simulink model "guitar2"  (Simulink 8.0)
settings: Solver=ode5  StartTime=0.0  StopTime=inf  FixedStep=0.001  RelTol=1e-3
libraries: simulink x4, xpclib x4, xpcnilib x4
settings Model: Creator=research account  LastModifiedBy=Admin  SimulationMode=external  BufferReuse=off
settings DataIOCC: SignalLoggingSaveFormat=ModelDataLogs
settings OptimizationCC: BlockReduction=off  OptimizeBlockIOStorage=off  BufferReuse=off  ExpressionFolding=off  LocalBlockOutputs=off
settings DebuggingCC: SingleTaskRateTransMsg=warning  FcnCallInpInsideContextMsg=UseLocalSettings  StrictBusMsg=Warning
settings HardwareCC: ProdIntDivRoundTo=Zero  ProdEndianess=LittleEndian  ProdHWDeviceType=Generic->32-bit x86 compatible
settings SFSimCC: SimParseCustomCode=off
settings RTWCC: SystemTargetFile=xpctarget.tlc  TemplateMakefile=xpc_default_tmf  Description=xPC Target  ProcessScript=xpctarget_make_rtw_hook  RTWCompilerOptimization=On
settings xpcTargetCC: TargetFcnLib=ansi_tfl_table_tmw.mat  CodeReplacementLibrary=XPC_BLAS  ParMdlRefBuildCompliant=on  ConcurrentExecutionCompliant=on  CombineSignalStateStructs=off  GRTInterface=on  xPCTaskExecutionProfile=off  xPCRL32EventNumber=5000  xpcObjCom=on  xPCLoadParamSetFile=off  xPCConcurrentTasks=off  xPCEnableSFAnimation=off

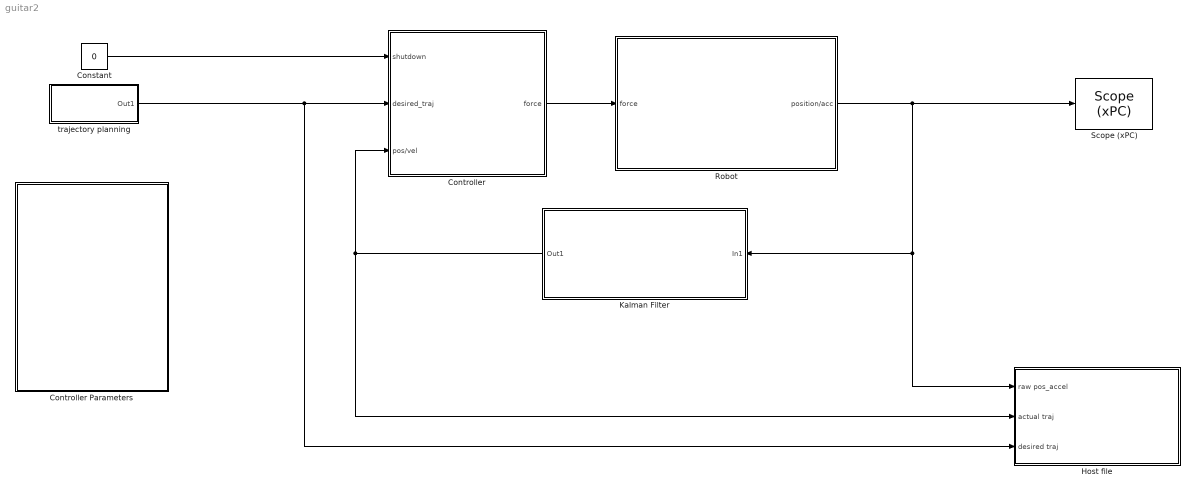
== system guitar2 ==
  Constant : Constant  Description=xPCTag(1) = onSwitch;  Value=0
  Controller : Subsystem
  Controller Parameters : Subsystem
      mask Display: disp('Controller Parameters')
  Host file : Subsystem
  Kalman Filter : Subsystem
  Robot : Subsystem
  "Scope (xPC) " : xpclib/Misc./Scope (xPC)   scopeno=1  scopetype=Target  autostart=on  viewmode=Graphical redraw  formatstr='%15.6f'  grid=on  ylimits=[0,0]  nosamples=500  noprepostsamples=0  interleave=1  triggermode=FreeRun  triggersignal=1  triggerlevel=0.0  triggerslope=Either  triggerscope=1  triggersample=0  filename=data.dat  mode=Lazy  writesize=512  autorestart=off  dynamicfilemode=off  maxwritefilesize=512*1024^2
  trajectory planning : Subsystem
  wires:
  Robot/1(position/acc) -> "Scope (xPC) "/1, Host file/1(raw pos_accel), Kalman Filter/1(In1)
  Constant/1 -> Controller/1(shutdown)
  Controller/1(force) -> Robot/1(force)
  trajectory planning/1(Out1) -> Controller/2(desired_traj), Host file/3(desired traj)
  Kalman Filter/1(Out1) -> Host file/2(actual traj), Controller/3(pos/vel)

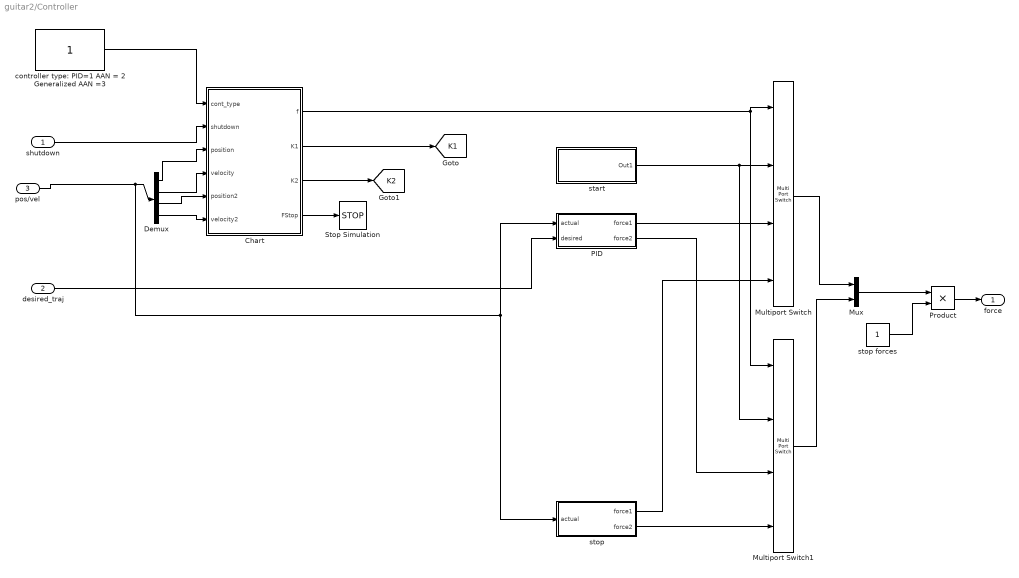
== system guitar2/Controller ==
  shutdown : Inport
  desired_traj : Inport  Port=2
  pos/vel : Inport  Port=3
  Chart : Stateflow chart  TreatAsAtomicUnit=on
  Demux : Demux
  Multiport Switch : MultiPortSwitch
  Multiport Switch1 : MultiPortSwitch
  Mux : Mux  Inputs=2
  PID : Subsystem
  Product : Product  RndMeth=Zero
  Stop Simulation : Stop
  controller type: PID=1 AAN = 2 Generalized AAN =3 : Constant
  start : Subsystem
  stop : Subsystem
  stop forces : Constant  Description=xPCTag(1) = stopForces;
  force : Outport
  tag scope: K1=global, K2=global
  wires:
  shutdown/1 -> Chart/2(shutdown)
  pos/vel/1 -> Demux/1, PID/1(actual), stop/1(actual)
  Demux/1 -> Chart/3(position)
  Demux/2 -> Chart/4(velocity)
  Chart/4(FStop) -> Stop Simulation/1
  controller type: PID=1 AAN = 2 Generalized AAN =3/1 -> Chart/1(cont_type)
  desired_traj/1 -> PID/2(desired)
  Chart/2(K1) -> [K1]
  Chart/3(K2) -> [K2]
  Demux/3 -> Chart/5(position2)
  Demux/4 -> Chart/6(velocity2)
  Mux/1 -> Product/1
  Product/1 -> force/1
  stop forces/1 -> Product/2
  Chart/1(f) -> Multiport Switch/1, Multiport Switch1/1
  start/1(Out1) -> Multiport Switch/2, Multiport Switch1/2
  PID/1(force1) -> Multiport Switch/3
  Multiport Switch/1 -> Mux/1
  PID/2(force2) -> Multiport Switch1/3
  stop/1(force1) -> Multiport Switch/4
  Multiport Switch1/1 -> Mux/2
  stop/2(force2) -> Multiport Switch1/4

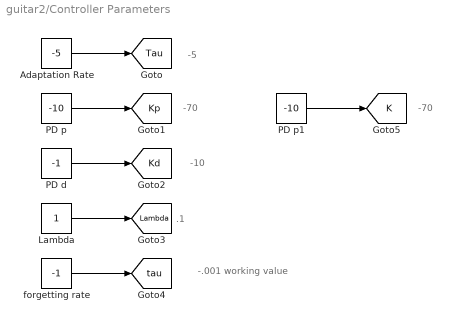
== system guitar2/Controller Parameters ==
  note: -.001 working value
  note: .1
  note: -10
  note: -70
  note: -5
  note: -70
  Adaptation Rate : Constant  Description=xPCTag(1)=learning_rate;  Value=-5
  Lambda : Constant
  PD d : Constant  Value=-1
  PD p : Constant  Value=-10
  PD p1 : Constant  Value=-10
  forgetting rate : Constant  Description=xPCTag(1)=forgetting_rate;  Value=-1
  tag scope: K=global, Kd=global, Kp=global, Lambda=global, Tau=global, tau=global
  wires:
  Adaptation Rate/1 -> [Tau]
  PD p/1 -> [Kp]
  PD d/1 -> [Kd]
  Lambda/1 -> [Lambda]
  forgetting rate/1 -> [tau]
  PD p1/1 -> [K]

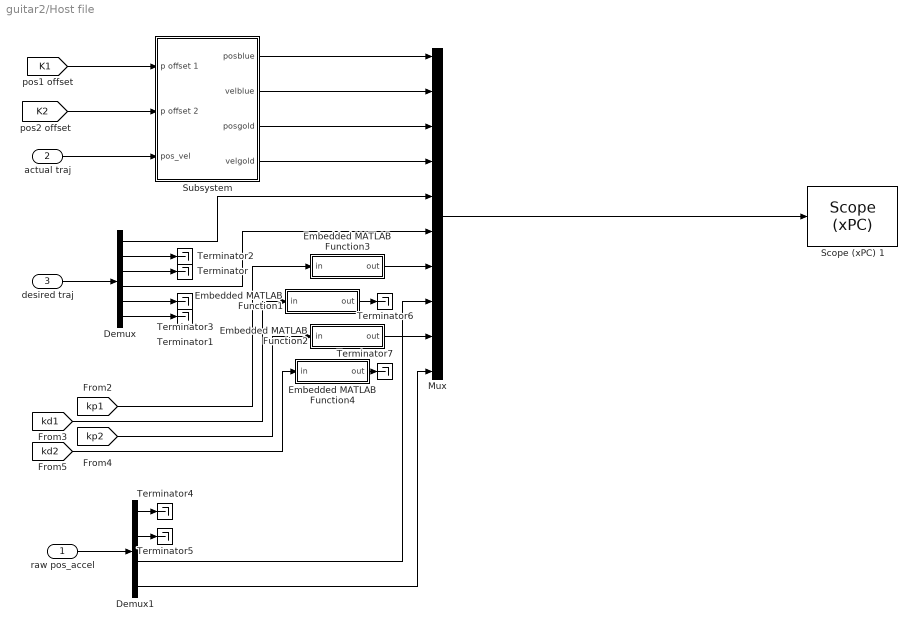
== system guitar2/Host file ==
  raw pos_accel : Inport
  actual traj : Inport  Port=2
  desired traj : Inport  Port=3
  Demux : Demux  Outputs=6
  Demux1 : Demux
  Embedded MATLAB Function1 : MATLAB Function  TreatAsAtomicUnit=on
  Embedded MATLAB Function2 : MATLAB Function  TreatAsAtomicUnit=on
  Embedded MATLAB Function3 : MATLAB Function  TreatAsAtomicUnit=on
  Embedded MATLAB Function4 : MATLAB Function  TreatAsAtomicUnit=on
  Mux : Mux  Inputs=10
  Scope (xPC) 1 : xpclib/Misc./Scope (xPC)   scopeno=3  scopetype=Host  autostart=on  viewmode=Graphical redraw  formatstr='%15.6f'  grid=on  ylimits=[0,0]  nosamples=500  noprepostsamples=0  interleave=1  triggermode=FreeRun  triggersignal=1  triggerlevel=0.0  triggerslope=Either  triggerscope=1  triggersample=0  filename=data.dat  mode=Lazy  writesize=512  autorestart=off  dynamicfilemode=off  maxwritefilesize=512*1024^2
  Subsystem : Subsystem
  Terminator{,1..7} (8 alike) : Terminator
  wires:
  desired traj/1 -> Demux/1
  Demux/3 -> Terminator/1
  Demux/6 -> Terminator1/1
  Demux/2 -> Terminator2/1
  Demux/5 -> Terminator3/1
  actual traj/1 -> Subsystem/3(pos_vel)
  [K1] -> Subsystem/1(p offset 1)
  [K2] -> Subsystem/2(p offset 2)
  Subsystem/1(posblue) -> Mux/1
  Subsystem/2(velblue) -> Mux/2
  Subsystem/3(posgold) -> Mux/3
  Subsystem/4(velgold) -> Mux/4
  Demux/1 -> Mux/5
  Demux/4 -> Mux/6
  [kp1] -> Embedded MATLAB Function3/1(in)
  [kd1] -> Embedded MATLAB Function1/1(in)
  [kp2] -> Embedded MATLAB Function2/1(in)
  [kd2] -> Embedded MATLAB Function4/1(in)
  Mux/1 -> Scope (xPC) 1/1
  Embedded MATLAB Function3/1(out) -> Mux/7
  Embedded MATLAB Function2/1(out) -> Mux/9
  raw pos_accel/1 -> Demux1/1
  Demux1/4 -> Mux/10
  Demux1/1 -> Terminator4/1
  Embedded MATLAB Function1/1(out) -> Terminator6/1
  Embedded MATLAB Function4/1(out) -> Terminator7/1
  Demux1/2 -> Terminator5/1
  Demux1/3 -> Mux/8

== system guitar2/Kalman Filter ==
  note: positions and velocities tagged here!
  In1 : Inport
  Demux : Demux
  Gain : Gain
  Mux : Mux  Inputs=2
  kalman1 : Subsystem
  kalman2 : Subsystem
  kalman3 : Subsystem
  kalman4 : Subsystem
  Out1 : Outport
  wires:
  Demux/1 -> kalman3/1(position)
  Demux/2 -> kalman4/1(position)
  Demux/3 -> kalman3/2(acc)
  Demux/4 -> kalman4/2(acc)
  In1/1 -> Demux/1
  kalman3/1(position/est_vel) -> Mux/1
  kalman4/1(position/est_vel) -> Mux/2
  Mux/1 -> Gain/1
  Gain/1 -> Out1/1

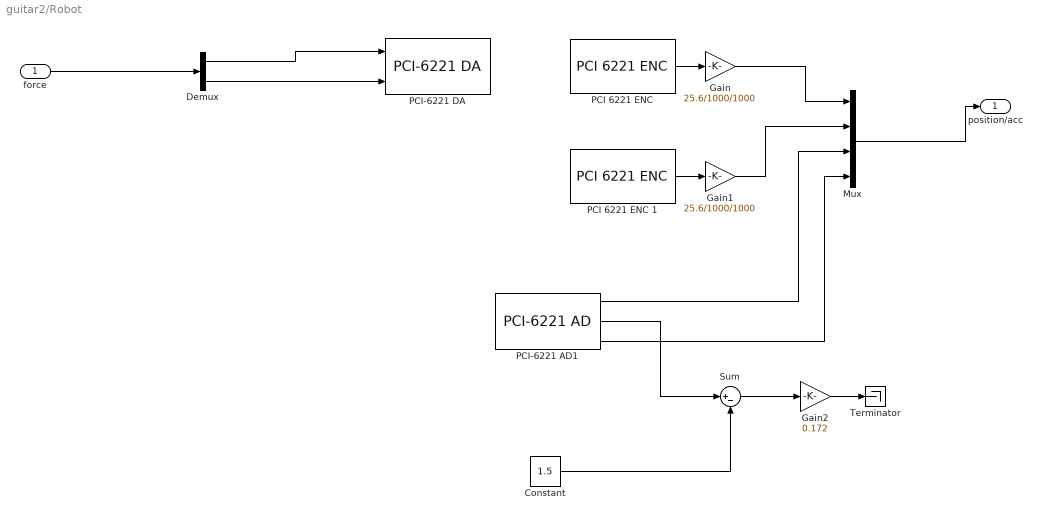
== system guitar2/Robot ==
  force : Inport
  Constant : Constant  Value=1.5
  Demux : Demux  Outputs=2
  Gain : Gain  Gain=25.6/1000/1000
  Gain1 : Gain  Gain=25.6/1000/1000
  Gain2 : Gain  Gain=0.172
  Mux : Mux
  "PCI 6221 ENC " : xpcnilib/Incremental Encoder/PCI 6221 ENC   channel=0  countMode=Quadrature Mode x4  initCount=0  reload=off  indexPhase=A low B low  filter=Minimum pulse width 125 nanoseconds  sampleTime=0.001  slot=-1
  PCI 6221 ENC 1 : xpcnilib/Incremental Encoder/PCI 6221 ENC   channel=1  countMode=Quadrature Mode x4  initCount=0  reload=off  indexPhase=A low B low  filter=Minimum pulse width 125 nanoseconds  sampleTime=0.001  slot=-1
  PCI-6221 AD1 : xpcnilib/A//D/M Series/PCI-6221 AD  channel=[1 2 3]  range=[10]  coupling=[0]  scantime=5e-6  sampletime=0.001  slot=-1
  PCI-6221 DA : xpcnilib/D//A/M Series/PCI-6221 DA  channel=[1 2]  reset=[1]  initValue=[0]  sampletime=0.001  slot=-1
  Sum : Sum  Inputs=|+-
  Terminator : Terminator
  position/acc : Outport
  wires:
  "PCI 6221 ENC "/1 -> Gain/1
  Gain/1 -> Mux/1
  Mux/1 -> position/acc/1
  Demux/1 -> PCI-6221 DA/1
  Demux/2 -> PCI-6221 DA/2
  force/1 -> Demux/1
  PCI 6221 ENC 1/1 -> Gain1/1
  Gain1/1 -> Mux/2
  PCI-6221 AD1/1 -> Mux/3
  PCI-6221 AD1/3 -> Mux/4
  PCI-6221 AD1/2 -> Sum/1
  Constant/1 -> Sum/2
  Sum/1 -> Gain2/1
  Gain2/1 -> Terminator/1

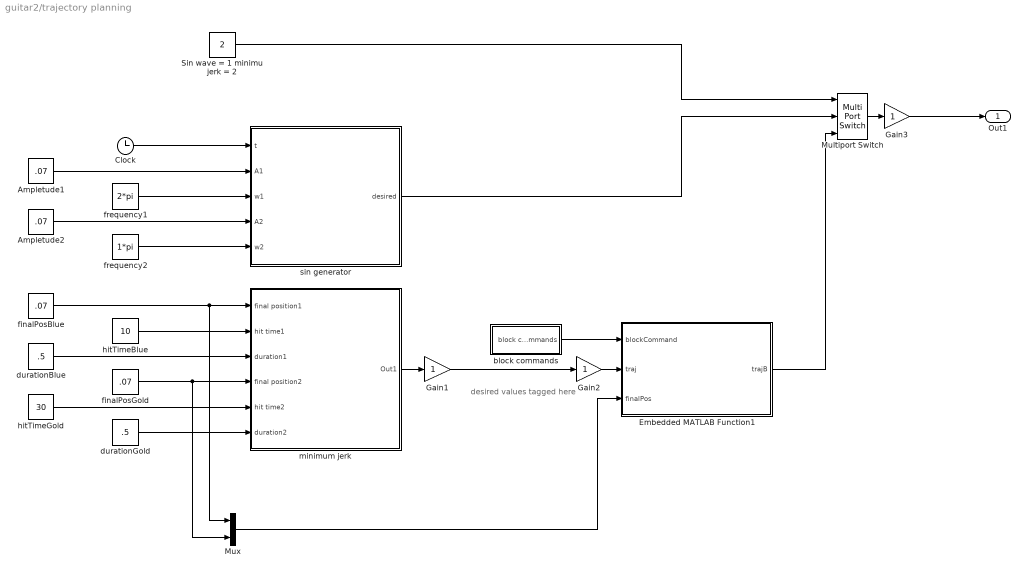
== system guitar2/trajectory planning ==
  note: desired values tagged here
  Ampletude1 : Constant  Value=.07
  Ampletude2 : Constant  Value=.07
  Clock : Clock
  Embedded MATLAB Function1 : MATLAB Function  TreatAsAtomicUnit=on
  Gain1 : Gain
  Gain2 : Gain
  Gain3 : Gain
  Multiport Switch : MultiPortSwitch  Inputs=2
  Mux : Mux  Inputs=2
  Sin wave = 1 minimu jerk = 2 : Constant  Value=2
  block commands : Subsystem
  durationBlue : Constant  Description=xPCTag(1) = durationBlue;  Value=.5
  durationGold : Constant  Description=xPCTag(1) = durationGold;  Value=.5
  finalPosBlue : Constant  Description=xPCTag(1) = finalPosBlue;  Value=.07
  finalPosGold : Constant  Description=xPCTag(1) = finalPosGold;  Value=.07
  frequency1 : Constant  Value=2*pi
  frequency2 : Constant  Value=1*pi
  hitTimeBlue : Constant  Description=xPCTag(1) = hitTimeBlue;  Value=10
  hitTimeGold : Constant  Description=xPCTag(1) = hitTimeGold;  Value=30
  minimum jerk : Subsystem
  sin generator : MATLAB Function  TreatAsAtomicUnit=on
  Out1 : Outport
  wires:
  Ampletude1/1 -> sin generator/2(A1)
  frequency1/1 -> sin generator/3(w1)
  Clock/1 -> sin generator/1(t)
  sin generator/1(desired) -> Multiport Switch/2
  Sin wave = 1 minimu jerk = 2/1 -> Multiport Switch/1
  Multiport Switch/1 -> Gain3/1
  Ampletude2/1 -> sin generator/4(A2)
  frequency2/1 -> sin generator/5(w2)
  finalPosBlue/1 -> minimum jerk/1(final position1), Mux/1
  hitTimeBlue/1 -> minimum jerk/2(hit time1)
  durationBlue/1 -> minimum jerk/3(duration1)
  finalPosGold/1 -> Mux/2, minimum jerk/4(final position2)
  hitTimeGold/1 -> minimum jerk/5(hit time2)
  durationGold/1 -> minimum jerk/6(duration2)
  minimum jerk/1(Out1) -> Gain1/1
  Embedded MATLAB Function1/1(trajB) -> Multiport Switch/3
  Mux/1 -> Embedded MATLAB Function1/3(finalPos)
  block commands/1(block commands) -> Embedded MATLAB Function1/1(blockCommand)
  Gain1/1 -> Gain2/1
  Gain2/1 -> Embedded MATLAB Function1/2(traj)
  Gain3/1 -> Out1/1

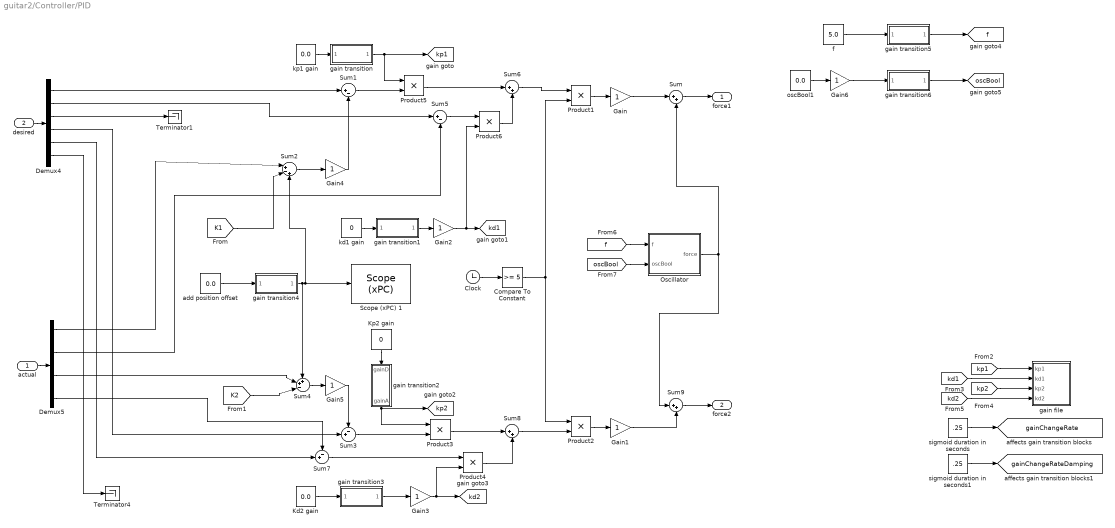
== system guitar2/Controller/PID ==
  actual : Inport
  desired : Inport  Port=2
  Clock : Clock
  Compare To Constant : simulink/Logic and Bit Operations/Compare To Constant  relop=>=  const=5  OutDataTypeStr=uint8
  Demux4 : Demux  Outputs=6
  Demux5 : Demux
  Gain{,1..6} (7 alike) : Gain
  Kd2 gain : Constant  Description=xPCTag(1)=Kd2;  Value=0.0
  Kp2 gain : Constant  Description=xPCTag(1)=Kp2;  Value=0
  Oscillator : Subsystem
  Product{1..6} (6 alike) : Product  RndMeth=Zero
  Scope (xPC) 1 : xpclib/Misc./Scope (xPC)   scopeno=6  scopetype=Target  autostart=on  viewmode=Graphical redraw  formatstr='%15.6f'  grid=on  ylimits=[0,0]  nosamples=500  noprepostsamples=0  interleave=1  triggermode=FreeRun  triggersignal=1  triggerlevel=0.0  triggerslope=Either  triggerscope=1  triggersample=0  filename=data.dat  mode=Lazy  writesize=512  autorestart=off  dynamicfilemode=off  maxwritefilesize=512*1024^2
  Sum{,6,8..9} (4 alike) : Sum  Inputs=|++
  Sum1 : Sum  Inputs=|+-
  Sum2 : Sum  Inputs=|+-+
  Sum3 : Sum  Inputs=-+|
  Sum4 : Sum  Inputs=++-|
  Sum5 : Sum  Inputs=|+-
  Sum7 : Sum  Inputs=-+|
  Terminator1 : Terminator
  Terminator4 : Terminator
  add position offset : Constant  Description=xPCTag(1)=posoffset;  Value=0.0
  f : Constant  Description=xPCTag(1)=f;  Value=5.0
  gain file : Subsystem
  gain transition : Subsystem
  gain transition1 : Subsystem
  gain transition2 : Subsystem
  gain transition3 : Subsystem
  gain transition4 : Subsystem
  gain transition5 : Subsystem
  gain transition6 : Subsystem
  kd1 gain : Constant  Description=xPCTag(1)=Kd1;  Value=0
  kp1 gain : Constant  Description=xPCTag(1)=Kp1;  Value=0.0
  oscBool1 : Constant  Description=xPCTag(1)=oscBool;  Value=0.0
  sigmoid duration in seconds : Constant  Description=xPCTag(1) = gcRate;  Value=.25
  sigmoid duration in seconds1 : Constant  Description=xPCTag(1) = gcRateDamping;  Value=.25
  force1 : Outport
  force2 : Outport  Port=2
  tag scope: f=global, gainChangeRate=global, gainChangeRateDamping=global, kd1=global, kd2=global, kp1=global, kp2=global, oscBool=global
  wires:
  Demux4/1 -> Sum1/1
  Demux4/2 -> Sum5/1
  Clock/1 -> Compare To Constant/1
  [K1] -> Sum2/2
  Sum2/1 -> Gain4/1
  Compare To Constant/1 -> Product1/2, Product2/1
  Sum1/1 -> Product5/2
  Product1/1 -> Gain/1
  Product2/1 -> Gain1/1
  desired/1 -> Demux4/1
  Demux4/3 -> Terminator1/1
  actual/1 -> Demux5/1
  Demux5/2 -> Sum5/2
  Demux5/4 -> Sum7/1
  Sum4/1 -> Gain5/1
  Demux4/4 -> Sum3/2
  Demux4/5 -> Sum7/2
  Demux4/6 -> Terminator4/1
  Sum3/1 -> Product3/2
  Gain/1 -> Sum/1
  Gain1/1 -> Sum9/2
  Product5/1 -> Sum6/1
  Product6/1 -> Sum6/2
  Sum6/1 -> Product1/1
  Sum7/1 -> Product4/1
  Product3/1 -> Sum8/1
  Product4/1 -> Sum8/2
  Sum8/1 -> Product2/2
  Kd2 gain/1 -> gain transition3/1(gainD)
  Sum5/1 -> Product6/1
  kd1 gain/1 -> gain transition1/1(gainD)
  Gain2/1 -> Product6/2, [kd1]
  Gain3/1 -> Product4/2, [kd2]
  Demux5/1 -> Sum2/1
  Demux5/3 -> Sum4/2
  add position offset/1 -> gain transition4/1(gainD)
  [K2] -> Sum4/3
  kp1 gain/1 -> gain transition/1(gainD)
  gain transition/1(gainA) -> Product5/1, [kp1]
  gain transition1/1(gainA) -> Gain2/1
  Kp2 gain/1 -> gain transition2/1(gainD)
  gain transition2/1(gainA) -> Product3/1, [kp2]
  gain transition3/1(gainA) -> Gain3/1
  sigmoid duration in seconds/1 -> [gainChangeRate]
  [kp1] -> gain file/1(kp1)
  [kd1] -> gain file/2(kd1)
  [kp2] -> gain file/3(kp2)
  [kd2] -> gain file/4(kd2)
  gain transition4/1(gainA) -> Scope (xPC) 1/1, Sum2/3, Sum4/1
  sigmoid duration in seconds1/1 -> [gainChangeRateDamping]
  Gain4/1 -> Sum1/2
  Gain5/1 -> Sum3/1
  [f] -> Oscillator/1(f)
  [oscBool] -> Oscillator/2(oscBool)
  Oscillator/1(force) -> Sum/2, Sum9/1
  Sum9/1 -> force2/1
  Sum/1 -> force1/1
  f/1 -> gain transition5/1(gainD)
  gain transition5/1(gainA) -> [f]
  oscBool1/1 -> Gain6/1
  gain transition6/1(gainA) -> [oscBool]
  Gain6/1 -> gain transition6/1(gainD)

== system guitar2/Controller/start ==
  Ramp : simulink/Sources/Ramp  slope=-.8  start=0  X0=0
  Saturation : Saturate  UpperLimit=2.5  LowerLimit=-2.5
  Out1 : Outport
  wires:
  Ramp/1 -> Saturation/1
  Saturation/1 -> Out1/1

== system guitar2/Controller/stop ==
  actual : Inport
  Demux : Demux
  Gain : Gain  Gain=-1
  Gain1 : Gain  Gain=-1
  Terminator : Terminator
  Terminator1 : Terminator
  force1 : Outport
  force2 : Outport  Port=2
  wires:
  Demux/1 -> Terminator/1
  actual/1 -> Demux/1
  Demux/2 -> Gain/1
  Gain/1 -> force1/1
  Demux/4 -> Gain1/1
  Gain1/1 -> force2/1
  Demux/3 -> Terminator1/1

== system guitar2/Host file/Subsystem ==
  p offset 1 : Inport
  p offset 2 : Inport  Port=2
  pos_vel : Inport  Port=3
  Demux1 : Demux
  Sum : Sum  Inputs=|-+
  Sum1 : Sum  Inputs=|-+
  posblue : Outport
  velblue : Outport  Port=2
  posgold : Outport  Port=3
  velgold : Outport  Port=4
  wires:
  Demux1/1 -> Sum/2
  Sum/1 -> posblue/1
  Demux1/3 -> Sum1/2
  Sum1/1 -> posgold/1
  p offset 1/1 -> Sum/1
  pos_vel/1 -> Demux1/1
  p offset 2/1 -> Sum1/1
  Demux1/2 -> velblue/1
  Demux1/4 -> velgold/1

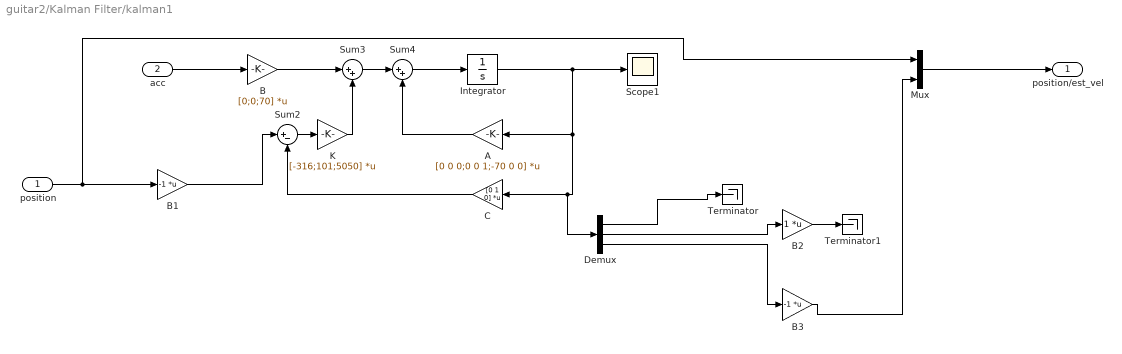
== system guitar2/Kalman Filter/kalman1 ==
  position : Inport
  acc : Inport  Port=2
  A : Gain  Gain=[0 0 0;0 0 1;-70 0 0]  Multiplication=Matrix(K*u)
  B : Gain  Gain=[0;0;70]  Multiplication=Matrix(K*u)
  B1 : Gain  Gain=-1  Multiplication=Matrix(K*u)
  B2 : Gain  Multiplication=Matrix(K*u)
  B3 : Gain  Gain=-1  Multiplication=Matrix(K*u)
  C : Gain  Gain=[0 1 0]  Multiplication=Matrix(K*u)
  Demux : Demux  Outputs=3
  Integrator : Integrator  InitialCondition=[1.5;0;0]
  K : Gain  Gain=[-316;101;5050]  Multiplication=Matrix(K*u)
  Mux : Mux  Inputs=2
  Scope1 : Scope
  Sum2 : Sum  Inputs=|+-
  Sum3 : Sum  Inputs=|++
  Sum4 : Sum  Inputs=|++
  Terminator : Terminator
  Terminator1 : Terminator
  position/est_vel : Outport
  wires:
  Integrator/1 -> A/1, C/1, Demux/1, Scope1/1
  C/1 -> Sum2/2
  Sum2/1 -> K/1
  B/1 -> Sum3/1
  K/1 -> Sum3/2
  Sum3/1 -> Sum4/1
  A/1 -> Sum4/2
  Sum4/1 -> Integrator/1
  Demux/2 -> B2/1
  Demux/3 -> B3/1
  Demux/1 -> Terminator/1
  B1/1 -> Sum2/1
  B3/1 -> Mux/2
  B2/1 -> Terminator1/1
  Mux/1 -> position/est_vel/1
  acc/1 -> B/1
  position/1 -> Mux/1, B1/1

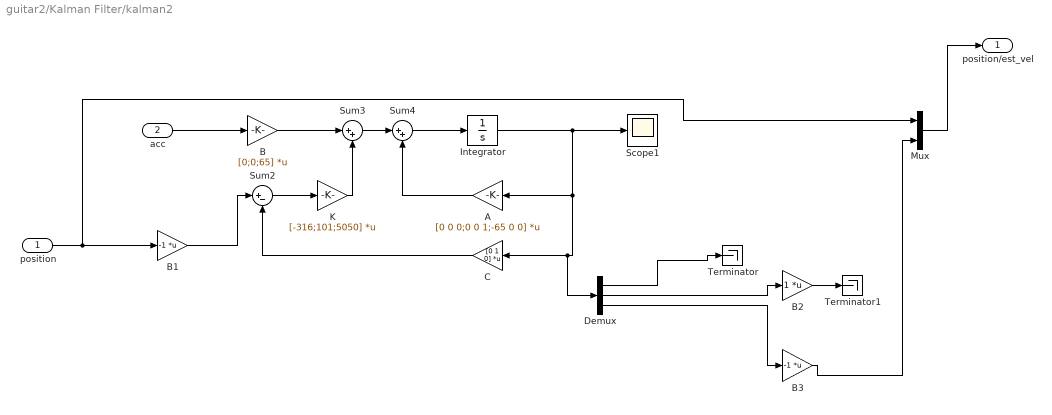
== system guitar2/Kalman Filter/kalman2 ==
  position : Inport
  acc : Inport  Port=2
  A : Gain  Gain=[0 0 0;0 0 1;-65 0 0]  Multiplication=Matrix(K*u)
  B : Gain  Gain=[0;0;65]  Multiplication=Matrix(K*u)
  B1 : Gain  Gain=-1  Multiplication=Matrix(K*u)
  B2 : Gain  Multiplication=Matrix(K*u)
  B3 : Gain  Gain=-1  Multiplication=Matrix(K*u)
  C : Gain  Gain=[0 1 0]  Multiplication=Matrix(K*u)
  Demux : Demux  Outputs=3
  Integrator : Integrator  InitialCondition=[1.5;0;0]
  K : Gain  Gain=[-316;101;5050]  Multiplication=Matrix(K*u)
  Mux : Mux  Inputs=2
  Scope1 : Scope
  Sum2 : Sum  Inputs=|+-
  Sum3 : Sum  Inputs=|++
  Sum4 : Sum  Inputs=|++
  Terminator : Terminator
  Terminator1 : Terminator
  position/est_vel : Outport
  wires:
  acc/1 -> B/1
  Mux/1 -> position/est_vel/1
  B2/1 -> Terminator1/1
  B3/1 -> Mux/2
  B1/1 -> Sum2/1
  Demux/1 -> Terminator/1
  Demux/3 -> B3/1
  Demux/2 -> B2/1
  Sum4/1 -> Integrator/1
  A/1 -> Sum4/2
  Sum3/1 -> Sum4/1
  K/1 -> Sum3/2
  B/1 -> Sum3/1
  Sum2/1 -> K/1
  C/1 -> Sum2/2
  Integrator/1 -> Scope1/1, Demux/1, C/1, A/1
  position/1 -> Mux/1, B1/1

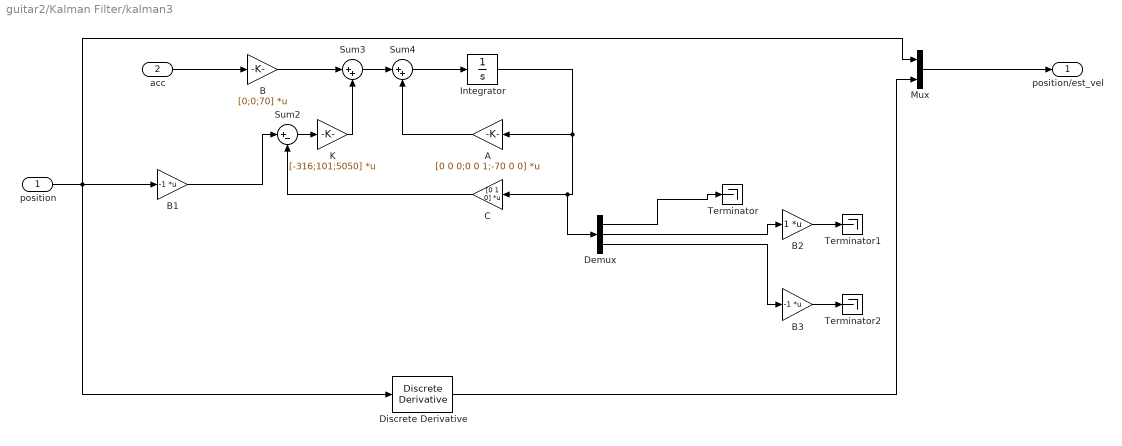
== system guitar2/Kalman Filter/kalman3 ==
  position : Inport
  acc : Inport  Port=2
  A : Gain  Gain=[0 0 0;0 0 1;-70 0 0]  Multiplication=Matrix(K*u)
  B : Gain  Gain=[0;0;70]  Multiplication=Matrix(K*u)
  B1 : Gain  Gain=-1  Multiplication=Matrix(K*u)
  B2 : Gain  Multiplication=Matrix(K*u)
  B3 : Gain  Gain=-1  Multiplication=Matrix(K*u)
  C : Gain  Gain=[0 1 0]  Multiplication=Matrix(K*u)
  Demux : Demux  Outputs=3
  Discrete Derivative : simulink/Discrete/Discrete Derivative  gainval=1.0  ICPrevScaledInput=0.0  InputProcessing=Inherited  OutMin=[]  OutMax=[]  OutDataType=fixdt(1, 16)  OutScaling=2^-10  DoSatur=off
  Integrator : Integrator  InitialCondition=[1.5;0;0]
  K : Gain  Gain=[-316;101;5050]  Multiplication=Matrix(K*u)
  Mux : Mux  Inputs=2
  Sum2 : Sum  Inputs=|+-
  Sum3 : Sum  Inputs=|++
  Sum4 : Sum  Inputs=|++
  Terminator : Terminator
  Terminator1 : Terminator
  Terminator2 : Terminator
  position/est_vel : Outport
  wires:
  Integrator/1 -> A/1, C/1, Demux/1
  C/1 -> Sum2/2
  Sum2/1 -> K/1
  B/1 -> Sum3/1
  K/1 -> Sum3/2
  Sum3/1 -> Sum4/1
  A/1 -> Sum4/2
  Sum4/1 -> Integrator/1
  Demux/2 -> B2/1
  Demux/3 -> B3/1
  Demux/1 -> Terminator/1
  B1/1 -> Sum2/1
  B2/1 -> Terminator1/1
  Mux/1 -> position/est_vel/1
  acc/1 -> B/1
  position/1 -> Discrete Derivative/1, Mux/1, B1/1
  Discrete Derivative/1 -> Mux/2
  B3/1 -> Terminator2/1

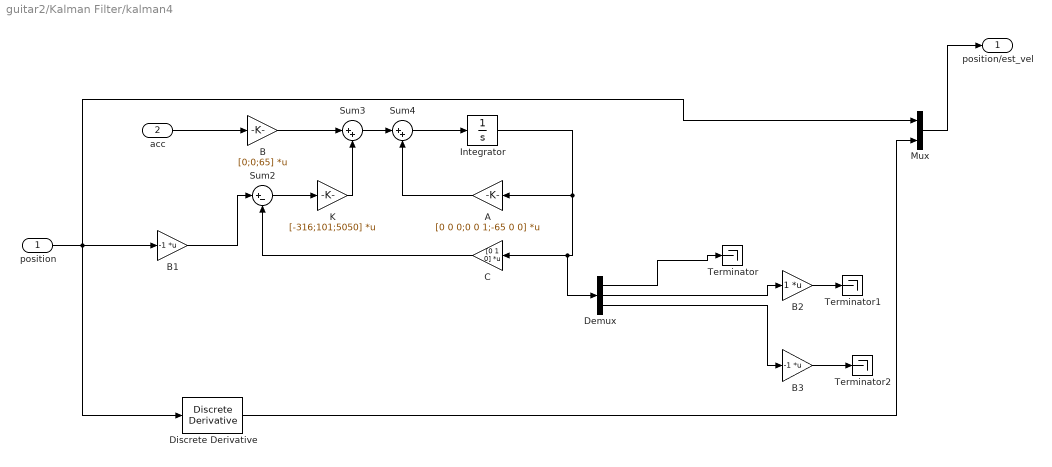
== system guitar2/Kalman Filter/kalman4 ==
  position : Inport
  acc : Inport  Port=2
  A : Gain  Gain=[0 0 0;0 0 1;-65 0 0]  Multiplication=Matrix(K*u)
  B : Gain  Gain=[0;0;65]  Multiplication=Matrix(K*u)
  B1 : Gain  Gain=-1  Multiplication=Matrix(K*u)
  B2 : Gain  Multiplication=Matrix(K*u)
  B3 : Gain  Gain=-1  Multiplication=Matrix(K*u)
  C : Gain  Gain=[0 1 0]  Multiplication=Matrix(K*u)
  Demux : Demux  Outputs=3
  Discrete Derivative : simulink/Discrete/Discrete Derivative  gainval=1.0  ICPrevScaledInput=0.0  InputProcessing=Inherited  OutMin=[]  OutMax=[]  OutDataType=fixdt(1, 16)  OutScaling=2^-10  DoSatur=off
  Integrator : Integrator  InitialCondition=[1.5;0;0]
  K : Gain  Gain=[-316;101;5050]  Multiplication=Matrix(K*u)
  Mux : Mux  Inputs=2
  Sum2 : Sum  Inputs=|+-
  Sum3 : Sum  Inputs=|++
  Sum4 : Sum  Inputs=|++
  Terminator : Terminator
  Terminator1 : Terminator
  Terminator2 : Terminator
  position/est_vel : Outport
  wires:
  acc/1 -> B/1
  Mux/1 -> position/est_vel/1
  B2/1 -> Terminator1/1
  B1/1 -> Sum2/1
  Demux/1 -> Terminator/1
  Demux/3 -> B3/1
  Demux/2 -> B2/1
  Sum4/1 -> Integrator/1
  A/1 -> Sum4/2
  Sum3/1 -> Sum4/1
  K/1 -> Sum3/2
  B/1 -> Sum3/1
  Sum2/1 -> K/1
  C/1 -> Sum2/2
  Integrator/1 -> Demux/1, C/1, A/1
  position/1 -> Discrete Derivative/1, Mux/1, B1/1
  Discrete Derivative/1 -> Mux/2
  B3/1 -> Terminator2/1

== system guitar2/trajectory planning/block commands ==
  Mux1 : Mux  Inputs=3
  block command blue : Constant  Description=xPCTag(1) = blockComBlue;  Value=0
  block command gold : Constant  Description=xPCTag(1) = blockComGold;  Value=0
  block fraction : Constant  Description=xPCTag(1) = blockThresh;  Value=.075
  block commands : Outport
  wires:
  block command blue/1 -> Mux1/1
  block command gold/1 -> Mux1/2
  Mux1/1 -> block commands/1
  block fraction/1 -> Mux1/3

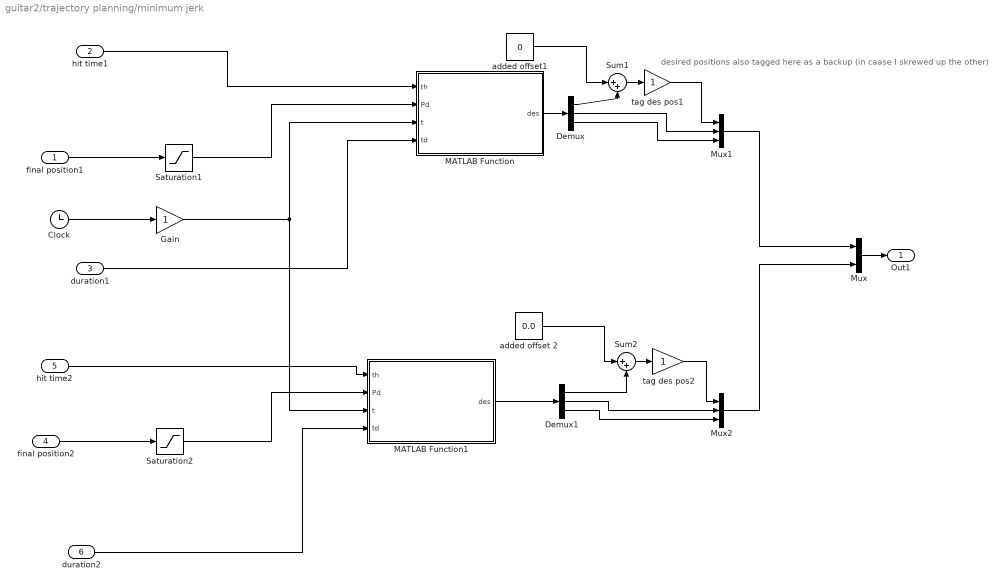
== system guitar2/trajectory planning/minimum jerk ==
  note: desired positions also tagged here as a backup (in caase I skrewed up the other)
  final position1 : Inport
  hit time1 : Inport  Port=2
  duration1 : Inport  Port=3
  final position2 : Inport  Port=4
  hit time2 : Inport  Port=5
  duration2 : Inport  Port=6
  Clock : Clock
  Demux : Demux  Outputs=3
  Demux1 : Demux  Outputs=3
  Gain : Gain
  MATLAB Function : MATLAB Function  TreatAsAtomicUnit=on
  MATLAB Function1 : MATLAB Function  TreatAsAtomicUnit=on
  Mux : Mux  Inputs=2
  Mux1 : Mux  Inputs=3
  Mux2 : Mux  Inputs=3
  Saturation1 : Saturate  UpperLimit=.17  LowerLimit=-10
  Saturation2 : Saturate  UpperLimit=.17  LowerLimit=-10
  Sum1 : Sum  Inputs=|++
  Sum2 : Sum  Inputs=|++
  added offset 2 : Constant  Description=xPCTag(1)=blockoffset2;  Value=0.0
  added offset1 : Constant  Description=xPCTag(1)=blockoffset1;  Value=0
  tag des pos1 : Gain
  tag des pos2 : Gain
  Out1 : Outport
  wires:
  final position1/1 -> Saturation1/1
  Saturation1/1 -> MATLAB Function/2(Pd)
  Clock/1 -> Gain/1
  hit time1/1 -> MATLAB Function/1(th)
  duration1/1 -> MATLAB Function/4(td)
  final position2/1 -> Saturation2/1
  hit time2/1 -> MATLAB Function1/1(th)
  Saturation2/1 -> MATLAB Function1/2(Pd)
  duration2/1 -> MATLAB Function1/4(td)
  Mux/1 -> Out1/1
  Gain/1 -> MATLAB Function/3(t), MATLAB Function1/3(t)
  MATLAB Function/1(des) -> Demux/1
  added offset1/1 -> Sum1/1
  Demux/1 -> Sum1/2
  Sum1/1 -> tag des pos1/1
  Demux/2 -> Mux1/2
  Demux/3 -> Mux1/3
  Mux1/1 -> Mux/1
  MATLAB Function1/1(des) -> Demux1/1
  added offset 2/1 -> Sum2/1
  Demux1/1 -> Sum2/2
  Sum2/1 -> tag des pos2/1
  Demux1/2 -> Mux2/2
  Demux1/3 -> Mux2/3
  Mux2/1 -> Mux/2
  tag des pos1/1 -> Mux1/1
  tag des pos2/1 -> Mux2/1

== system guitar2/Controller/PID/Oscillator ==
  f : Inport
  oscBool : Inport  Port=2
  Clock : Clock
  MATLAB Function : MATLAB Function  TreatAsAtomicUnit=on
  force : Outport
  wires:
  Clock/1 -> MATLAB Function/1(t)
  f/1 -> MATLAB Function/2(f)
  oscBool/1 -> MATLAB Function/3(oscBool)
  MATLAB Function/1(y) -> force/1

== system guitar2/Controller/PID/gain file ==
  kp1 : Inport
  kd1 : Inport  Port=2
  kp2 : Inport  Port=3
  kd2 : Inport  Port=4
  Mux : Mux
  "Scope (xPC) " : xpclib/Misc./Scope (xPC)   scopeno=2  scopetype=File  autostart=on  viewmode=Graphical redraw  formatstr='%15.6f'  grid=on  ylimits=[0,0]  nosamples=10000  noprepostsamples=0  interleave=1  triggermode=FreeRun  triggersignal=1  triggerlevel=0.0  triggerslope=Either  triggerscope=1  triggersample=0  filename=data.dat  mode=Lazy  writesize=512  autorestart=on  dynamicfilemode=off  maxwritefilesize=512*1024^2
  file readable outputs : MATLAB Function  TreatAsAtomicUnit=on
  wires:
  Mux/1 -> file readable outputs/1(u)
  file readable outputs/1(y) -> "Scope (xPC) "/1
  kp1/1 -> Mux/1
  kd1/1 -> Mux/2
  kp2/1 -> Mux/3
  kd2/1 -> Mux/4

== system guitar2/Controller/PID/gain transition ==
  gainD : Inport
  Memory : Memory  X0=zeros(1,4)
  gainramp : MATLAB Function  TreatAsAtomicUnit=on
  gainA : Outport
  wires:
  Memory/1 -> gainramp/3(state)
  gainramp/2(state1) -> Memory/1
  [gainChangeRate] -> gainramp/1(tr)
  gainramp/1(val) -> gainA/1
  gainD/1 -> gainramp/2(valD)

== system guitar2/Controller/PID/gain transition1 ==
  gainD : Inport
  Memory : Memory  X0=zeros(1,4)
  gainramp : MATLAB Function  TreatAsAtomicUnit=on
  gainA : Outport
  wires:
  Memory/1 -> gainramp/3(state)
  gainramp/2(state1) -> Memory/1
  [gainChangeRate] -> gainramp/1(tr)
  gainramp/1(val) -> gainA/1
  gainD/1 -> gainramp/2(valD)

== system guitar2/Controller/PID/gain transition2 ==
  gainD : Inport
  Memory : Memory  X0=zeros(1,4)
  gainramp : MATLAB Function  TreatAsAtomicUnit=on
  gainA : Outport
  wires:
  Memory/1 -> gainramp/3(state)
  gainramp/2(state1) -> Memory/1
  gainramp/1(val) -> gainA/1
  gainD/1 -> gainramp/2(valD)
  [gainChangeRateDamping] -> gainramp/1(tr)

== system guitar2/Controller/PID/gain transition3 ==
  gainD : Inport
  Memory : Memory  X0=zeros(1,4)
  gainramp : MATLAB Function  TreatAsAtomicUnit=on
  gainA : Outport
  wires:
  Memory/1 -> gainramp/3(state)
  gainramp/2(state1) -> Memory/1
  [gainChangeRate] -> gainramp/1(tr)
  gainramp/1(val) -> gainA/1
  gainD/1 -> gainramp/2(valD)

== system guitar2/Controller/PID/gain transition4 ==
  gainD : Inport
  Constant : Constant  Value=.75
  Memory : Memory  X0=zeros(1,4)
  gainramp : MATLAB Function  TreatAsAtomicUnit=on
  gainA : Outport
  wires:
  Memory/1 -> gainramp/3(state)
  gainramp/2(state1) -> Memory/1
  Constant/1 -> gainramp/1(tr)
  gainramp/1(val) -> gainA/1
  gainD/1 -> gainramp/2(valD)

== system guitar2/Controller/PID/gain transition5 ==
  gainD : Inport
  Constant : Constant
  Memory : Memory  X0=zeros(1,4)
  gainramp : MATLAB Function  TreatAsAtomicUnit=on
  gainA : Outport
  wires:
  Memory/1 -> gainramp/3(state)
  gainramp/2(state1) -> Memory/1
  gainramp/1(val) -> gainA/1
  gainD/1 -> gainramp/2(valD)
  Constant/1 -> gainramp/1(tr)

== system guitar2/Controller/PID/gain transition6 ==
  gainD : Inport
  Constant : Constant
  Memory : Memory  X0=zeros(1,4)
  gainramp : MATLAB Function  TreatAsAtomicUnit=on
  gainA : Outport
  wires:
  Memory/1 -> gainramp/3(state)
  gainramp/2(state1) -> Memory/1
  Constant/1 -> gainramp/1(tr)
  gainramp/1(val) -> gainA/1
  gainD/1 -> gainramp/2(valD)

== stateflow chart Controller/Chart ==
  state Start
    du: f=1; FStop=0;
    du: K1=position; K2=position2;
  state pid
    du: f=2;
  state assist
    du: f=3;
  state generalized
    du: f=4;
  state Stop
    en: TT=t;
    du: f=5; FStop=(t-TT >1)*abs(velocity)<.01*abs(velocity2)<.01;
  (default) -> Start
  Start -> generalized [order 4] : [t>5 & cont_type==3]
  Start -> assist [order 3] : [t>5 & cont_type==2]
  Start -> Stop [order 1] : [shutdown==1]
  Start -> pid [order 2] : [ t>5 & cont_type==1]
  generalized -> Stop : [t>2000 | velocity>2 | velocity2>2 | shutdown==1]
  assist -> Stop : [t>2000 | velocity>2 | velocity2>2 | shutdown == 1]
  pid -> Stop : [t>2000 | velocity>2 | velocity2>2 |shutdown == 1]
  data: cont_type input double; shutdown input double; position input double; velocity input double; f output double; K1 output double; TT local double; position2 input double; velocity2 input double; K2 output double; FStop output double

== matlab function trajectory planning/sin generator ==
  data: t input double; desired output double; A1 input double; w1 input double; A2 input double; w2 input double
function desired = fcn(t,A1,w1,A2,w2)
%#codegen

desired = [A1*sin(w1*t-pi/2-5*w1)+A1;A1*w1*cos(w1*t-pi/2-5*w1);-A1*w1^2*sin(w1*t-pi/2-5*w1);...
    A2*sin(w2*t-pi/2-5*w2)+A2;A2*w2*cos(w2*t-pi/2-5*w2);-A2*w2^2*sin(w2*t-pi/2-5*w2)];

== matlab function trajectory planning/minimum jerk/MATLAB Function ==
  data: th input double; des output double; Pd input double; t input double; td input double
function des = fcn(th, Pd, t, td)
%#codegen
if t > th-td && t<=th
T=t-(th-td);
des=[(10*Pd*T^3)/td^3 - (15*Pd*T^4)/td^4 + (6*Pd*T^5)/td^5;...
(30*Pd*T^2)/td^3 - (60*Pd*T^3)/td^4 + (30*Pd*T^4)/td^5;...
(120*Pd*T^3)/td^5 - (180*Pd*T^2)/td^4 + (60*Pd*T)/td^3];
elseif th<t && t<th+td
T=t-th;
des=[Pd - (10*Pd*T^3)/td^3 + (15*Pd*T^4)/td^4 - (6*Pd*T^5)/td^5;...
(60*Pd*T^3)/td^4 - (30*Pd*T^2)/td^3 - (30*Pd*T^4)/td^5;...
(180*Pd*T^2)/td^4 - (120*Pd*T^3)/td^5 - (60*Pd*T)/td^3];
else
des=[0;0;0];
end

== matlab function Controller/PID/gain file/file readable outputs ==
  data: u input double; y output double
function y = inisout(u)
%#eml

y = u;

== matlab function Controller/PID/gain transition/gainramp ==
  data: val output double; tr input double; valD input double; state1 output double; state input double
% state contains [valD_,val_,Ro_,t_]
function [val,state1] = fcn(tr,valD,state)
%#eml

% first we need to check if they have changed the desired Value
if ~ (valD == state(1))
    state(1) = valD;
    state(4) = 0;
    state(3) = state(1) - state(2);
end

t = state(4);
Ro = state(3);

if ((t <= tr) && (tr~=0))
    Rd = Ro - Ro*(10*(t)^3/(tr)^3 - 15*(t)^4/(tr)^4 + 6*(t)^5/(tr)^5);
else
    Rd = 0;
end

val = state(1) - Rd;
state(2) = val;
state(4) = t + .001;
state1 = state;

== matlab function trajectory planning/minimum jerk/MATLAB Function1 ==
  data: th input double; des output double; Pd input double; t input double; td input double
function des = fcn(th, Pd, t, td)
%#codegen
if t > th-td && t<=th
T=t-(th-td);
des=[(10*Pd*T^3)/td^3 - (15*Pd*T^4)/td^4 + (6*Pd*T^5)/td^5;...
(30*Pd*T^2)/td^3 - (60*Pd*T^3)/td^4 + (30*Pd*T^4)/td^5;...
(120*Pd*T^3)/td^5 - (180*Pd*T^2)/td^4 + (60*Pd*T)/td^3];
elseif th<t && t<th+td
T=t-th;
des=[Pd - (10*Pd*T^3)/td^3 + (15*Pd*T^4)/td^4 - (6*Pd*T^5)/td^5;...
(60*Pd*T^3)/td^4 - (30*Pd*T^2)/td^3 - (30*Pd*T^4)/td^5;...
(180*Pd*T^2)/td^4 - (120*Pd*T^3)/td^5 - (60*Pd*T)/td^3];
else
des=[0;0;0];
end

== matlab function Controller/PID/gain transition1/gainramp ==
  data: val output double; tr input double; valD input double; state1 output double; state input double
% state contains [valD_,val_,Ro_,t_]
function [val,state1] = fcn(tr,valD,state)
%#eml

% first we need to check if they have changed the desired Value
if ~ (valD == state(1))
    state(1) = valD;
    state(4) = 0;
    state(3) = state(1) - state(2);
end

t = state(4);
Ro = state(3);

if ((t <= tr) && (tr~=0))
    Rd = Ro - Ro*(10*(t)^3/(tr)^3 - 15*(t)^4/(tr)^4 + 6*(t)^5/(tr)^5);
else
    Rd = 0;
end

val = state(1) - Rd;
state(2) = val;
state(4) = t + .001;
state1 = state;

== matlab function Controller/PID/gain transition2/gainramp ==
  data: val output double; tr input double; valD input double; state1 output double; state input double
% state contains [valD_,val_,Ro_,t_]
function [val,state1] = fcn(tr,valD,state)
%#eml

% first we need to check if they have changed the desired Value
if ~ (valD == state(1))
    state(1) = valD;
    state(4) = 0;
    state(3) = state(1) - state(2);
end

t = state(4);
Ro = state(3);

if ((t <= tr) && (tr~=0))
    Rd = Ro - Ro*(10*(t)^3/(tr)^3 - 15*(t)^4/(tr)^4 + 6*(t)^5/(tr)^5);
else
    Rd = 0;
end

val = state(1) - Rd;
state(2) = val;
state(4) = t + .001;
state1 = state;

== matlab function Controller/PID/gain transition3/gainramp ==
  data: val output double; tr input double; valD input double; state1 output double; state input double
% state contains [valD_,val_,Ro_,t_]
function [val,state1] = fcn(tr,valD,state)
%#eml

% first we need to check if they have changed the desired Value
if ~ (valD == state(1))
    state(1) = valD;
    state(4) = 0;
    state(3) = state(1) - state(2);
end

t = state(4);
Ro = state(3);

if ((t <= tr) && (tr~=0))
    Rd = Ro - Ro*(10*(t)^3/(tr)^3 - 15*(t)^4/(tr)^4 + 6*(t)^5/(tr)^5);
else
    Rd = 0;
end

val = state(1) - Rd;
state(2) = val;
state(4) = t + .001;
state1 = state;

== matlab function Controller/PID/gain transition4/gainramp ==
  data: val output double; tr input double; valD input double; state1 output double; state input double
% state contains [valD_,val_,Ro_,t_]
function [val,state1] = fcn(tr,valD,state)
%#eml

% first we need to check if they have changed the desired Value
if ~ (valD == state(1))
    state(1) = valD;
    state(4) = 0;
    state(3) = state(1) - state(2);
end

t = state(4);
Ro = state(3);

if ((t <= tr) && (tr~=0))
    Rd = Ro - Ro*(10*(t)^3/(tr)^3 - 15*(t)^4/(tr)^4 + 6*(t)^5/(tr)^5);
else
    Rd = 0;
end

val = state(1) - Rd;
state(2) = val;
state(4) = t + .001;
state1 = state;

== matlab function Controller/PID/Oscillator/MATLAB Function ==
  data: t input double; f input double; oscBool input double; y output double
function y = fcn(t,f,oscBool)
%#codegen

% inputs
% t = time
% f = frequency
% oscillateBool turns oscillator on or off using a ramp (0->1)

%oscillator
y = oscBool*sin(f*2*pi*t);

end

== matlab function Host file/Embedded MATLAB Function1 ==
  data: in input double; out output double
function out = dn(in)
%#eml
% the output just follows tyhe input. We need to do this in order to read the signal into the dang scope
out = in;

== matlab function Host file/Embedded MATLAB Function2 ==
  data: in input double; out output double
function out = dn(in)
%#eml
% the output just follows tyhe input. We need to do this in order to read the signal into the dang scope
out = in;

== matlab function Host file/Embedded MATLAB Function4 ==
  data: in input double; out output double
function out = dn(in)
%#eml
% the output just follows tyhe input. We need to do this in order to read the signal into the dang scope
out = in;

== matlab function Host file/Embedded MATLAB Function3 ==
  data: in input double; out output double
function out = dn(in)
%#eml
% the output just follows tyhe input. We need to do this in order to read the signal into the dang scope
out = in;

== matlab function trajectory planning/Embedded MATLAB Function1 ==
  data: blockCommand input double; traj input double; finalPos input double; trajB output double
% this function will alow us to check how much the subjects are moving
% during their blocked notes. If a note is designated as a blocked note
% (by the blockSignal input) then this function will try to clamp the
% subjects in place during a short period of their movement. We will try
% to hold them when their velocity should be at it's greatest. 

% let's make this simpler. just cut the tips off of the blocked notes.

function trajB = noteBlocker(blockCommand, traj, finalPos)
%#eml

blockSignalB = blockCommand(1);
blockSignalG= blockCommand(2);
blockThresh = blockCommand(3);
finalPosB = finalPos(1);
finalPosG = finalPos(2);

% if we are blocking the blue finger
if ((blockSignalB == 1))
    if (traj(1) > blockThresh) 
        traj(1) = blockThresh;
        traj(2) = 0;
        traj(3) = 0;
    end
end

% if we are blocking the blue finger
if (blockSignalG == 1) 
    if (traj(4) > blockThresh)
        traj(4) = blockThresh;
        traj(5) = 0;
        traj(6) = 0;
    end
end

% shat should do it.

trajB = traj;

== matlab function Controller/PID/gain transition5/gainramp ==
  data: val output double; tr input double; valD input double; state1 output double; state input double
% state contains [valD_,val_,Ro_,t_]
function [val,state1] = fcn(tr,valD,state)
%#eml

% first we need to check if they have changed the desired Value
if ~ (valD == state(1))
    state(1) = valD;
    state(4) = 0;
    state(3) = state(1) - state(2);
end

t = state(4);
Ro = state(3);

if ((t <= tr) && (tr~=0))
    Rd = Ro - Ro*(10*(t)^3/(tr)^3 - 15*(t)^4/(tr)^4 + 6*(t)^5/(tr)^5);
else
    Rd = 0;
end

val = state(1) - Rd;
state(2) = val;
state(4) = t + .001;
state1 = state;

== matlab function Controller/PID/gain transition6/gainramp ==
  data: val output double; tr input double; valD input double; state1 output double; state input double
% state contains [valD_,val_,Ro_,t_]
function [val,state1] = fcn(tr,valD,state)
%#eml

% first we need to check if they have changed the desired Value
if ~ (valD == state(1))
    state(1) = valD;
    state(4) = 0;
    state(3) = state(1) - state(2);
end

t = state(4);
Ro = state(3);

if ((t <= tr) && (tr~=0))
    Rd = Ro - Ro*(10*(t)^3/(tr)^3 - 15*(t)^4/(tr)^4 + 6*(t)^5/(tr)^5);
else
    Rd = 0;
end

val = state(1) - Rd;
state(2) = val;
state(4) = t + .001;
state1 = state;
